simulink library "Driveline_Axle2_A1_L2_R2_A1Diff"  (R2026a)
settings: Solver=VariableStepAuto
undefined symbols (not defined in the file): ShaftA1, ShaftL2, ShaftR2
libraries: Driveshaft_ShaftsAll x4, fl_lib x3, sdl_lib x3, nesl_utility x2, Differential_Systems x1, sm_lib x1
Description:
  | Component of Simscape Vehicle Templates Library
  | 
  | Copyright 2018-2026 The MathWorks, Inc.
settings Model: Creator=smiller  LastModifiedBy=smiller

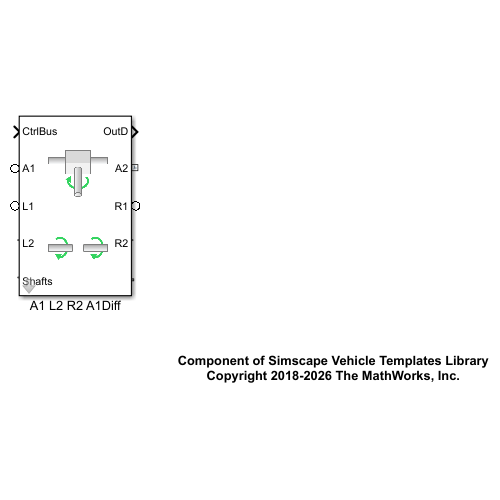
[thumbnail: Simulink's stored preview of the top-level diagram]
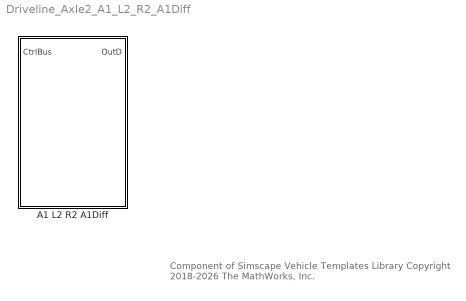
== system Driveline_Axle2_A1_L2_R2_A1Diff ==
  note: Component of Simscape Vehicle Templates Library
      | Copyright 2018-2026 The MathWorks, Inc.
  A1 L2 R2 A1Diff : Subsystem  Tag=PublishSubsystem  VariantControl=IndepFRDiffFDiffR  mask(Driveline, Two-Axle, Three Input Shaft){InitTriggerDropdown=0}
      mask prompts: InitTriggerDropdown "Initialization Trigger Dropdown"
      mask help: Models two-axle driveline with three separate shafts. A differential connects the front wheels, the other shafts are connected independently to the rear wheels.
      mask init:
      | curblk = gcb;
      | 
      | % Trigger Mask Initialization for 
      | % variant subsystems below this level
      | sm_car_lib_maskInitTrigger(curblk)
      mask TypeOptions InitTriggerDropdown: 0 | 1
      mask Display: image('sm_car_vehicle_driveline_axle2_a1_l2_r2_a1diff_IMAGE.png');

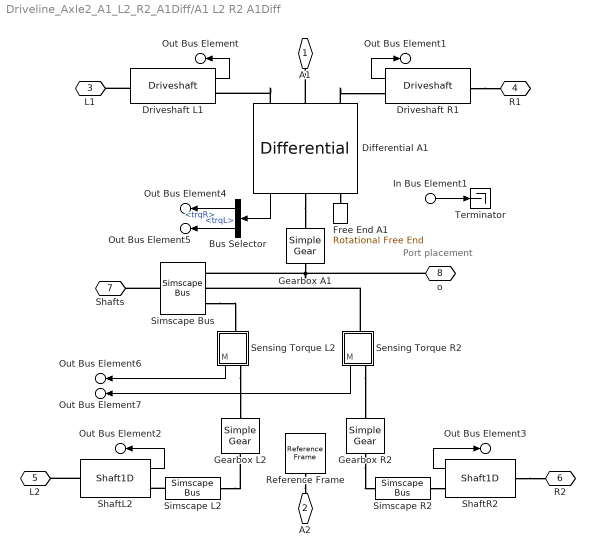
== system Driveline_Axle2_A1_L2_R2_A1Diff/A1 L2 R2 A1Diff ==
  note: Port
      | placement
  In Bus Element1 : Inport  PortName=CtrlBus
  Bus Selector : BusSelector  OutputSignals=trqR,trqL
  Differential A1 : Differential_Systems/Differential  VariantControl=Variant1  Differential=Driveline.DifferentialA1  VariantLabel=Driveline.DifferentialA1.class.Value  InitTriggerDropdown=0
      settings: AttributesFormatString=%<ActiveVariant>
  Driveshaft L1 : Driveshaft_ShaftsAll/Driveshaft  VariantControl=Variant1  popup_leftRight=Left  Driveshaft=Driveline.DriveshaftL1  VariantLabel=Driveline.DriveshaftL1.class.Value  InitTriggerDropdown=0
      settings: AttributesFormatString=%<ActiveVariant>
  Driveshaft R1 : Driveshaft_ShaftsAll/Driveshaft  VariantControl=Variant1  popup_leftRight=Right  Driveshaft=Driveline.DriveshaftR1  VariantLabel=Driveline.DriveshaftR1.class.Value  InitTriggerDropdown=0
      settings: AttributesFormatString=%<ActiveVariant>
  Free End A1 : fl_lib/Mechanical/Rotational Elements/Rotational Free End  w_specify=off  w_priority=None  w=0 rad/s  w_nominal_specify=off  w_nominal_value=1  w_nominal_unit=rad/s
  Gearbox A1 : sdl_lib/Gears/Simple Gear  ratio=Driveline.GearboxA1.ratio.Value  rotation_direction=3-2*(1)  friction_model=1  T_noload=0.1 N*m  T_nom=5 N*m  efficiency_nom=0.8  efficiency=0.8  temperature_TLU=[280, 300, 320] K  load_TLU=[1, 5, 10] N*m  efficiency_TLU=[.95, .9, .85]  efficiency_TLU2=[.85, .8, .75; .95, .9, .85; .85, .8, .7]  w_thr=0.01 rad/s  pwr_thr=0.001 W  enable_backlash=false  hardstop_model=simscape.enum.hardstop.smooth  backlash_distance=1e-3 mm  r_base=0.1 m  transition=1e-4 mm  backlash_stiffness=1e7 N/m  backlash_damping=1e6 N*s/m  coeff_rest=0  v_tol=0.001 m/s  f_tol=0 N  tau=0.1 s  mu_visc=[0, 0] N*m/(rad/s)  thermal_mass=50 J/K  temperature_specify=off  temperature_priority=High  temperature=300 K  temperature_nominal_specify=off  temperature_nominal_value=1  temperature_nominal_unit=K  x_backlash_specify=off  x_backlash_priority=None  x_backlash=0 mm  x_backlash_nominal_specify=off  x_backlash_nominal_value=1  x_backlash_nominal_unit=mm  f_hardstop_specify=off  f_hardstop_priority=None  f_hardstop=0 N  f_hardstop_nominal_specify=off  f_hardstop_nominal_value=1  f_hardstop_nominal_unit=N  v_backlash_specify=off  v_backlash_priority=None  v_backlash=0 m/s  v_backlash_nominal_specify=off  v_backlash_nominal_value=1  v_backlash_nominal_unit=m/s
  Gearbox L2 : sdl_lib/Gears/Simple Gear  ratio=Driveline.GearboxL2.ratio.Value  rotation_direction=3-2*(1)  friction_model=1  T_noload=0.1 N*m  T_nom=5 N*m  efficiency_nom=0.8  efficiency=0.8  temperature_TLU=[280, 300, 320] K  load_TLU=[1, 5, 10] N*m  efficiency_TLU=[.95, .9, .85]  efficiency_TLU2=[.85, .8, .75; .95, .9, .85; .85, .8, .7]  w_thr=0.01 rad/s  pwr_thr=0.001 W  enable_backlash=false  hardstop_model=simscape.enum.hardstop.smooth  backlash_distance=1e-3 mm  r_base=0.1 m  transition=1e-4 mm  backlash_stiffness=1e7 N/m  backlash_damping=1e6 N*s/m  coeff_rest=0  v_tol=0.001 m/s  f_tol=0 N  tau=0.1 s  mu_visc=[0, 0] N*m/(rad/s)  thermal_mass=50 J/K  temperature_specify=off  temperature_priority=High  temperature=300 K  temperature_nominal_specify=off  temperature_nominal_value=1  temperature_nominal_unit=K  x_backlash_specify=off  x_backlash_priority=None  x_backlash=0 mm  x_backlash_nominal_specify=off  x_backlash_nominal_value=1  x_backlash_nominal_unit=mm  f_hardstop_specify=off  f_hardstop_priority=None  f_hardstop=0 N  f_hardstop_nominal_specify=off  f_hardstop_nominal_value=1  f_hardstop_nominal_unit=N  v_backlash_specify=off  v_backlash_priority=None  v_backlash=0 m/s  v_backlash_nominal_specify=off  v_backlash_nominal_value=1  v_backlash_nominal_unit=m/s
  Gearbox R2 : sdl_lib/Gears/Simple Gear  ratio=Driveline.GearboxR2.ratio.Value  rotation_direction=3-2*(1)  friction_model=1  T_noload=0.1 N*m  T_nom=5 N*m  efficiency_nom=0.8  efficiency=0.8  temperature_TLU=[280, 300, 320] K  load_TLU=[1, 5, 10] N*m  efficiency_TLU=[.95, .9, .85]  efficiency_TLU2=[.85, .8, .75; .95, .9, .85; .85, .8, .7]  w_thr=0.01 rad/s  pwr_thr=0.001 W  enable_backlash=false  hardstop_model=simscape.enum.hardstop.smooth  backlash_distance=1e-3 mm  r_base=0.1 m  transition=1e-4 mm  backlash_stiffness=1e7 N/m  backlash_damping=1e6 N*s/m  coeff_rest=0  v_tol=0.001 m/s  f_tol=0 N  tau=0.1 s  mu_visc=[0, 0] N*m/(rad/s)  thermal_mass=50 J/K  temperature_specify=off  temperature_priority=High  temperature=300 K  temperature_nominal_specify=off  temperature_nominal_value=1  temperature_nominal_unit=K  x_backlash_specify=off  x_backlash_priority=None  x_backlash=0 mm  x_backlash_nominal_specify=off  x_backlash_nominal_value=1  x_backlash_nominal_unit=mm  f_hardstop_specify=off  f_hardstop_priority=None  f_hardstop=0 N  f_hardstop_nominal_specify=off  f_hardstop_nominal_value=1  f_hardstop_nominal_unit=N  v_backlash_specify=off  v_backlash_priority=None  v_backlash=0 m/s  v_backlash_nominal_specify=off  v_backlash_nominal_value=1  v_backlash_nominal_unit=m/s
  Reference Frame : sm_lib/Frames and Transforms/Reference Frame
  Sensing Torque L2 : Subsystem
  Sensing Torque R2 : Subsystem
  ShaftL2 : Driveshaft_ShaftsAll/Shaft1D  VariantControl=Shaft1D
  ShaftR2 : Driveshaft_ShaftsAll/Shaft1D  VariantControl=Shaft1D
  Simscape Bus : SimscapeBus  HierarchyStrings=ShaftA1;ShaftR2;ShaftL2
  Simscape L2 : SimscapeBus  HierarchyStrings=Shaft1D
  Simscape R2 : SimscapeBus  HierarchyStrings=Shaft1D
  Terminator : Terminator
  A1 : PMIOPort  Side=Left
  A2 : PMIOPort  Port=2  Side=Right
  L1 : PMIOPort  Port=3  Side=Left
  R1 : PMIOPort  Port=4  Side=Right
  L2 : PMIOPort  Port=5  Side=Left
  R2 : PMIOPort  Port=6  Side=Right
  Shafts : PMIOPort  Port=7  Side=Left
  o : PMIOPort  Port=8  Side=Right
  Out Bus Element6 : Outport  VectorParamsAs1DForOutWhenUnconnected=off  PortName=OutD  Element=MDriveshaftL2
  Out Bus Element7 : Outport  VectorParamsAs1DForOutWhenUnconnected=off  PortName=OutD  Element=MDriveshaftR2
  Out Bus Element4 : Outport  VectorParamsAs1DForOutWhenUnconnected=off  PortName=OutD  Element=MDriveshaftR1
  Out Bus Element5 : Outport  VectorParamsAs1DForOutWhenUnconnected=off  PortName=OutD  Element=MDriveshaftL1
  Out Bus Element : Outport  VectorParamsAs1DForOutWhenUnconnected=off  PortName=OutD  Element=anDriveshaftL1
  Out Bus Element1 : Outport  VectorParamsAs1DForOutWhenUnconnected=off  PortName=OutD  Element=anDriveshaftR1
  Out Bus Element2 : Outport  VectorParamsAs1DForOutWhenUnconnected=off  PortName=OutD  Element=anDriveshaftL2
  Out Bus Element3 : Outport  VectorParamsAs1DForOutWhenUnconnected=off  PortName=OutD  Element=anDriveshaftR2
  wires:
  In Bus Element1/1 -> Terminator/1
  Bus Selector/2 -> Out Bus Element5/1  "<trqL>"
  Bus Selector/1 -> Out Bus Element4/1  "<trqR>"
  Sensing Torque L2/1(M) -> Out Bus Element6/1
  Sensing Torque R2/1(M) -> Out Bus Element7/1
  Differential A1/1 -> Bus Selector/1
  ShaftR2/1 -> Out Bus Element3/1
  ShaftL2/1 -> Out Bus Element2/1
  Driveshaft L1/1 -> Out Bus Element/1
  Driveshaft R1/1 -> Out Bus Element1/1
  connections:
  Simscape Bus/RConn1 -- Shafts/RConn1
  Gearbox R2/RConn1 -- Simscape R2/LConn1
  Simscape R2/RConn1 -- ShaftR2/RConn1
  ShaftL2/LConn1 -- L2/RConn1
  ShaftR2/LConn1 -- R2/RConn1
  Differential A1/RConn1 -- Gearbox A1/RConn1
  Reference Frame/RConn1 -- A2/RConn1
  Differential A1/LConn2 -- A1/RConn1
  Driveshaft L1/LConn1 -- L1/RConn1
  Driveshaft R1/LConn1 -- R1/RConn1
  Differential A1/LConn3 -- Driveshaft R1/RConn1
  Differential A1/LConn1 -- Driveshaft L1/RConn1
  Differential A1/RConn2 -- Free End A1/LConn1
  Gearbox A1/LConn1 -- o/RConn1 -- Simscape Bus/LConn1
  Sensing Torque R2/LConn1 -- Simscape Bus/LConn2
  Simscape L2/RConn1 -- ShaftL2/RConn1
  Simscape L2/LConn1 -- Gearbox L2/RConn1
  Simscape Bus/LConn3 -- Sensing Torque L2/LConn1
  Sensing Torque L2/RConn1 -- Gearbox L2/LConn1
  Sensing Torque R2/RConn1 -- Gearbox R2/LConn1

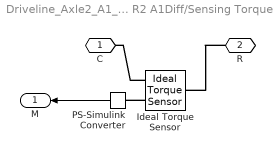
== system Driveline_Axle2_A1_L2_R2_A1Diff/A1 L2 R2 A1Diff/Sensing Torque L2 ==
  Ideal Torque Sensor : fl_lib/Mechanical/Mechanical Sensors/Ideal Torque Sensor
  PS-Simulink Converter : nesl_utility/PS-Simulink Converter  PhysicalDomain=network_engine_domain  SubClassName=ps_output  LeftPortType=input  RightPortType=output  PseudoPeriodic=off  Frequencies=[]  VectorFormat=1-D array  Unit=N*m  AffineConversion=off
  C : PMIOPort  Side=Right
  R : PMIOPort  Port=2  Side=Left
  M : Outport  VectorParamsAs1DForOutWhenUnconnected=off
  wires:
  PS-Simulink Converter/1 -> M/1
  connections:
  Ideal Torque Sensor/RConn1 -- C/RConn1
  R/RConn1 -- Ideal Torque Sensor/LConn1
  Ideal Torque Sensor/RConn2 -- PS-Simulink Converter/LConn1

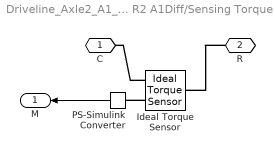
== system Driveline_Axle2_A1_L2_R2_A1Diff/A1 L2 R2 A1Diff/Sensing Torque R2 ==
  Ideal Torque Sensor : fl_lib/Mechanical/Mechanical Sensors/Ideal Torque Sensor
  PS-Simulink Converter : nesl_utility/PS-Simulink Converter  PhysicalDomain=network_engine_domain  SubClassName=ps_output  LeftPortType=input  RightPortType=output  PseudoPeriodic=off  Frequencies=[]  VectorFormat=1-D array  Unit=N*m  AffineConversion=off
  C : PMIOPort  Side=Right
  R : PMIOPort  Port=2  Side=Left
  M : Outport  VectorParamsAs1DForOutWhenUnconnected=off
  wires:
  PS-Simulink Converter/1 -> M/1
  connections:
  Ideal Torque Sensor/RConn2 -- PS-Simulink Converter/LConn1
  R/RConn1 -- Ideal Torque Sensor/LConn1
  Ideal Torque Sensor/RConn1 -- C/RConn1
